simulink model "car_model_5_28_2023"  (R2022b)
settings: Solver=VariableStepAuto  StartTime=0.0  StopTime=15  RelTol=1e-3
values from neighbouring files (symbols this model uses):
  dZ = 0.295    [Startup.m]
  F0z = [0 0]    [Startup.m]
  phi = 45    [Startup.m]
  X = Reference_Signals.Chassis_Position.X.Data(:)    [Simulation_Data_Parse.m]    (also in Vehicle_Sim_Parse.m = Chassis_Signals.InertFrm.Cg.Disp.X.Data(:))
  Y = Reference_Signals.Chassis_Position.Y.Data(:)    [Simulation_Data_Parse.m]    (also in Vehicle_Sim_Parse.m = Chassis_Signals.InertFrm.Cg.Disp.Y.Data(:))
undefined symbols (not defined in the file or in its folder): chassis, DiscIntNeverNeededParam, driver, IMU_accel, IMU_gyro, IMU_mag, powertrain, psi, sensor, sim, sus, suspension, theta, trn, tvs, veh, VEH, whl, Xdot, Ydot, Z, Zdot
libraries: fl_lib x53, nesl_utility x15, vehdynlibtire x10, vehdynlibsuspension x8, EngineCoolingComponents_lib x5, autolibutils x5, sharedtransform x5, dspstat3 x2, simulink x2, slpidlib x2, shared6dof x2, sensorgpslib x1
(part 6 of 9)

== system car_model_5_28_2023/Vehicle Model/Suspension/MacPherson Suspension/Wheel  Adapter ==
  Wheels : Inport
  Bus Selector : BusSelector  OutputSignals=SuspFrame.Fx,SuspFrame.Fy
  Bus Selector1 : BusSelector  OutputSignals=SuspFrame.Re
  Bus Selector2 : BusSelector  OutputSignals=SuspFrame.Mx,SuspFrame.My,SuspFrame.Mz
  Bus Selector3 : BusSelector  OutputSignals=SuspFrame.z,SuspFrame.zdot
  Matrix Concatenate : Concatenate  NumInputs=3  Mode=Multidimensional array
  Reshape{,1..7} (8 alike) : Reshape  OutputDimensionality=Row vector (2-D)
  WhlFx : Outport  VectorParamsAs1DForOutWhenUnconnected=off
  WhlFy : Outport  Port=2  VectorParamsAs1DForOutWhenUnconnected=off
  z : Outport  Port=3  VectorParamsAs1DForOutWhenUnconnected=off
  zdot : Outport  Port=4  VectorParamsAs1DForOutWhenUnconnected=off
  M : Outport  Port=5  VectorParamsAs1DForOutWhenUnconnected=off
  Re : Outport  Port=6  VectorParamsAs1DForOutWhenUnconnected=off
  wires:
  Reshape7/1 -> WhlFy/1
  Reshape6/1 -> WhlFx/1
  Bus Selector/1 -> Reshape6/1  "<Fx>"
  Bus Selector/2 -> Reshape7/1  "<Fy>"
  Bus Selector3/1 -> Reshape/1  "<z>"
  Wheels/1 -> Bus Selector1/1, Bus Selector2/1, Bus Selector3/1, Bus Selector/1
  Bus Selector3/2 -> Reshape2/1  "<zdot>"
  Reshape2/1 -> zdot/1  "zdot"
  Bus Selector1/1 -> Reshape1/1  "<Re>"
  Reshape1/1 -> Re/1  "Re"
  Bus Selector2/1 -> Reshape3/1  "<Mx>"
  Bus Selector2/2 -> Reshape4/1  "<My>"
  Bus Selector2/3 -> Reshape5/1  "<Mz>"
  Reshape3/1 -> Matrix Concatenate/1
  Reshape4/1 -> Matrix Concatenate/2
  Reshape5/1 -> Matrix Concatenate/3
  Matrix Concatenate/1 -> M/1  "M"
  Reshape/1 -> z/1  "z"

== system car_model_5_28_2023/Vehicle Model/Suspension/Mapped Suspension/Steer Rate Adapter ==
  Veh : Inport
  Add : Sum
  Bus Selector3 : BusSelector  OutputSignals=BdyFrm.Cg.AngVel.r
  Constant : Constant  Value=zeros(1,4)
  Matrix Concatenate : Concatenate  NumInputs=3  Mode=Multidimensional array
  Matrix Concatenate1 : Concatenate  NumInputs=3  Mode=Multidimensional array
  Reshape2 : Reshape  OutputDimensionality=Row vector (2-D)
  Reshape3 : Reshape  OutputDimensionality=Row vector (2-D)
  Reshape4 : Reshape  OutputDimensionality=Row vector (2-D)
  Selector3 : Selector  InputPortWidth=1  IndexOptions=Index vector (dialog)  Indices=[1 1 1 1]  OutputSizes=1
  SteerRates : Constant  Value=zeros(1,4)
  AngVel : Outport  VectorParamsAs1DForOutWhenUnconnected=off
  wires:
  Reshape2/1 -> Matrix Concatenate1/1, Matrix Concatenate1/3, Matrix Concatenate1/2
  Constant/1 -> Reshape3/1
  Selector3/1 -> Reshape4/1
  Bus Selector3/1 -> Selector3/1  "<r>"
  Matrix Concatenate/1 -> Add/2
  SteerRates/1 -> Reshape2/1
  Reshape4/1 -> Matrix Concatenate/3
  Reshape3/1 -> Matrix Concatenate/2, Matrix Concatenate/1
  Matrix Concatenate1/1 -> Add/1
  Veh/1 -> Bus Selector3/1
  Add/1 -> AngVel/1  "AngVel"

== system car_model_5_28_2023/Vehicle Model/Suspension/Mapped Suspension/Vehicle Adapter ==
  Veh : Inport
  Bus Creator3 : BusCreator  Inputs=2
  Bus Selector1 : BusSelector  OutputSignals=InertFrm.FrntAxl.Lft.Disp.X,InertFrm.FrntAxl.Lft.Disp.Y,InertFrm.FrntAxl.Lft.Disp.Z,InertFrm.FrntAxl.Rght.Disp.X,InertFrm.FrntAxl.Rght.Disp.Y,InertFrm.FrntAxl.Rght.Disp.Z,InertFrm.RearAxl.Lft.Disp.X,InertFrm.RearAxl.Lft.Disp.Y,InertFrm.RearAxl.Lft.Disp.Z,InertFrm.RearAxl.Rght.Disp.X,InertFrm.RearAxl.Rght.Disp.Y,InertFrm.RearAxl.Rght.Disp.Z
  Bus Selector2 : BusSelector  OutputSignals=BdyFrm.FrntAxl.Lft.Vel.xdot,BdyFrm.FrntAxl.Lft.Vel.ydot,BdyFrm.FrntAxl.Lft.Vel.zdot,BdyFrm.FrntAxl.Rght.Vel.xdot,BdyFrm.FrntAxl.Rght.Vel.ydot,BdyFrm.FrntAxl.Rght.Vel.zdot,BdyFrm.RearAxl.Lft.Vel.xdot,BdyFrm.RearAxl.Lft.Vel.ydot,BdyFrm.RearAxl.Lft.Vel.zdot,BdyFrm.RearAxl.Rght.Vel.xdot,BdyFrm.RearAxl.Rght.Vel.ydot,BdyFrm.RearAxl.Rght.Vel.zdot
  Bus Selector3 : BusSelector  OutputSignals=InertFrm.FrntAxl.Lft.Vel.Xdot,InertFrm.FrntAxl.Lft.Vel.Ydot,InertFrm.FrntAxl.Lft.Vel.Zdot,InertFrm.FrntAxl.Rght.Vel.Xdot,InertFrm.FrntAxl.Rght.Vel.Ydot,InertFrm.FrntAxl.Rght.Vel.Zdot,InertFrm.RearAxl.Lft.Vel.Xdot,InertFrm.RearAxl.Lft.Vel.Ydot,InertFrm.RearAxl.Lft.Vel.Zdot,InertFrm.RearAxl.Rght.Vel.Xdot,InertFrm.RearAxl.Rght.Vel.Ydot,InertFrm.RearAxl.Rght.Vel.Zdot
  Inertial Frame CG to Axle Offset : Constant  Value=[zeros(2,4);dZ*ones(1,4)]
  Mux1 : Mux  Inputs=12
  Mux2 : Mux  Inputs=12
  Mux3 : Mux  Inputs=12
  Reshape : Reshape  OutputDimensionality=Customize  OutputDimensions=[3,4]
  Reshape1 : Reshape  OutputDimensionality=Customize  OutputDimensions=[3,4]
  Reshape2 : Reshape  OutputDimensionality=Customize  OutputDimensions=[3,4]
  Sum : Sum  Inputs=|+-
  VehSusp : Outport  VectorParamsAs1DForOutWhenUnconnected=off
  VehVbody : Outport  Port=2  VectorParamsAs1DForOutWhenUnconnected=off
  wires:
  Veh/1 -> Bus Selector3/1, Bus Selector2/1, Bus Selector1/1
  Reshape2/1 -> VehVbody/1  "V"
  Bus Creator3/1 -> VehSusp/1  "Veh"
  Reshape/1 -> Sum/1
  Bus Selector1/1 -> Mux2/1  "<X>"
  Bus Selector1/2 -> Mux2/2  "<Y>"
  Bus Selector1/3 -> Mux2/3  "<Z>"
  Bus Selector1/4 -> Mux2/4  "<X>"
  Bus Selector1/5 -> Mux2/5  "<Y>"
  Bus Selector1/6 -> Mux2/6  "<Z>"
  Bus Selector1/7 -> Mux2/7  "<X>"
  Bus Selector1/8 -> Mux2/8  "<Y>"
  Bus Selector1/9 -> Mux2/9  "<Z>"
  Bus Selector1/10 -> Mux2/10  "<X>"
  Bus Selector1/11 -> Mux2/11  "<Y>"
  Bus Selector1/12 -> Mux2/12  "<Z>"
  Bus Selector2/1 -> Mux1/1  "<xdot>"
  Bus Selector2/2 -> Mux1/2  "<ydot>"
  Bus Selector2/3 -> Mux1/3  "<zdot>"
  Bus Selector2/4 -> Mux1/4  "<xdot>"
  Bus Selector2/5 -> Mux1/5  "<ydot>"
  Bus Selector2/6 -> Mux1/6  "<zdot>"
  Bus Selector2/7 -> Mux1/7  "<xdot>"
  Bus Selector2/8 -> Mux1/8  "<ydot>"
  Bus Selector2/9 -> Mux1/9  "<zdot>"
  Bus Selector2/10 -> Mux1/10  "<xdot>"
  Bus Selector2/11 -> Mux1/11  "<ydot>"
  Bus Selector2/12 -> Mux1/12  "<zdot>"
  Mux1/1 -> Reshape2/1
  Mux2/1 -> Reshape/1
  Inertial Frame CG to Axle Offset/1 -> Sum/2
  Sum/1 -> Bus Creator3/1  "P"
  Mux3/1 -> Reshape1/1
  Bus Selector3/12 -> Mux3/12  "<Zdot>"
  Bus Selector3/11 -> Mux3/11  "<Ydot>"
  Bus Selector3/10 -> Mux3/10  "<Xdot>"
  Bus Selector3/9 -> Mux3/9  "<Zdot>"
  Bus Selector3/8 -> Mux3/8  "<Ydot>"
  Bus Selector3/7 -> Mux3/7  "<Xdot>"
  Bus Selector3/6 -> Mux3/6  "<Zdot>"
  Bus Selector3/5 -> Mux3/5  "<Ydot>"
  Bus Selector3/4 -> Mux3/4  "<Xdot>"
  Bus Selector3/3 -> Mux3/3  "<Zdot>"
  Bus Selector3/2 -> Mux3/2  "<Ydot>"
  Bus Selector3/1 -> Mux3/1  "<Xdot>"
  Reshape1/1 -> Bus Creator3/2  "V"

== system car_model_5_28_2023/Vehicle Model/Suspension/Mapped Suspension/Wheel  Adapter ==
  Wheels : Inport
  Bus Selector : BusSelector  OutputSignals=SuspFrame.Fx,SuspFrame.Fy
  Bus Selector1 : BusSelector  OutputSignals=SuspFrame.Re
  Bus Selector2 : BusSelector  OutputSignals=SuspFrame.Mx,SuspFrame.My,SuspFrame.Mz
  Bus Selector3 : BusSelector  OutputSignals=SuspFrame.z,SuspFrame.zdot
  Matrix Concatenate : Concatenate  NumInputs=3  Mode=Multidimensional array
  Reshape{,1..7} (8 alike) : Reshape  OutputDimensionality=Row vector (2-D)
  WhlFx : Outport  VectorParamsAs1DForOutWhenUnconnected=off
  WhlFy : Outport  Port=2  VectorParamsAs1DForOutWhenUnconnected=off
  z : Outport  Port=3  VectorParamsAs1DForOutWhenUnconnected=off
  zdot : Outport  Port=4  VectorParamsAs1DForOutWhenUnconnected=off
  M : Outport  Port=5  VectorParamsAs1DForOutWhenUnconnected=off
  Re : Outport  Port=6  VectorParamsAs1DForOutWhenUnconnected=off
  wires:
  Reshape7/1 -> WhlFy/1
  Reshape6/1 -> WhlFx/1
  Bus Selector/1 -> Reshape6/1  "<Fx>"
  Bus Selector/2 -> Reshape7/1  "<Fy>"
  Bus Selector3/1 -> Reshape/1  "<z>"
  Wheels/1 -> Bus Selector1/1, Bus Selector2/1, Bus Selector3/1, Bus Selector/1
  Bus Selector3/2 -> Reshape2/1  "<zdot>"
  Reshape2/1 -> zdot/1  "zdot"
  Bus Selector1/1 -> Reshape1/1  "<Re>"
  Reshape1/1 -> Re/1  "Re"
  Bus Selector2/1 -> Reshape3/1  "<Mx>"
  Bus Selector2/2 -> Reshape4/1  "<My>"
  Bus Selector2/3 -> Reshape5/1  "<Mz>"
  Reshape3/1 -> Matrix Concatenate/1
  Reshape4/1 -> Matrix Concatenate/2
  Reshape5/1 -> Matrix Concatenate/3
  Matrix Concatenate/1 -> M/1  "M"
  Reshape/1 -> z/1  "z"

== system car_model_5_28_2023/Vehicle Model/Vehicle/6DOF/Suspension to Chasiss Transforms ==
  VehFdbk : Inport
  Suspension : Inport  Port=2
  Add : Sum  Inputs=+-
  Add1 : Sum
  Bus Selector : BusSelector  OutputSignals=BdyFrm.Cg.Vel.xdot
  Bus Selector1 : BusSelector  OutputSignals=BdyFrm.Cg.DCM
  Bus Selector2 : BusSelector  OutputSignals=BdyFrm.Cg.Acc.xddot,BdyFrm.Cg.Vel.ydot,BdyFrm.Cg.AngVel.r,BdyFrm.Cg.Acc.yddot,BdyFrm.Cg.Vel.xdot,BdyFrm.Cg.AngVel.r
  Bus Selector3 : BusSelector  OutputSignals=Whl.z,Veh.F,Veh.M
  Bus Selector4 : BusSelector  OutputSignals=InertFrm.Cg.Ang.phi,InertFrm.Cg.Ang.theta,InertFrm.Cg.Ang.psi  OutputAsBus=on
  Bus Selector6 : BusSelector  OutputSignals=InertFrm.Geom.Disp.X,InertFrm.Geom.Disp.Y,InertFrm.Geom.Disp.Z  OutputAsBus=on
  Bus to Vector3 : BusToVector
  Bus to Vector5 : BusToVector
  Bushings : autolibutils/Cont LPF  wc=40*pi  AbsoluteTolerance=auto  aMode=2
  Downforce : MATLAB Function  TreatAsAtomicUnit=on
  Estimated Unsprung Mass Orientation : MATLAB Function  TreatAsAtomicUnit=on  mask{trackW=mean(2.*chassis.geometry.s), wheelB=sum(chassis.geometry.l)}
      mask prompts: trackW "Vehicle track width, trackW [m]:"; wheelB "Vehicle wheelbase, wheelB [m]:"
      mask help: This block converts wheel ground height information into estimates of vehicle pitch, roll angles and vertical height in order to help in the visualization 3DOF based simulations with changes in terrain. Note that the resulting signals are only used as a visualization aid and do not account for the physical affects of the vehicle interacting with variable terrain or changes in orientation.
  Product : Product
  Product1 : Product
  Sum : Sum  Inputs=|++
  Susp2Body : Subsystem
  Terminator6 : Terminator
  Unary Minus : UnaryMinus
  Unsprung Masses : Gain  Gain=sum(chassis.mass.m_unsprung)  Multiplication=Matrix(u*K)
  Vector Concatenate : Concatenate
  Vector Concatenate1 : Concatenate
  Vertical : Constant  Value=0
  FsB : Outport
  MsB : Outport  Port=2
  Fext : Outport  Port=3
  wires:
  Bus Selector6/1 -> Bus to Vector5/1
  Bus Selector3/2 -> Susp2Body/4(Fs)  "<F>"
  VehFdbk/1 -> Bus Selector2/1, Bus Selector/1, Bus Selector1/1, Bus Selector6/1, Bus Selector4/1
  Bus Selector3/3 -> Susp2Body/5(Ms)  "<M>"
  Bus to Vector3/1 -> Estimated Unsprung Mass Orientation/1(angleIn), Susp2Body/2(VehAng)
  Bus Selector1/1 -> Susp2Body/1(DCM)  "<DCM>"
  Bus to Vector5/1 -> Estimated Unsprung Mass Orientation/2(GemoXYZIn)
  Suspension/1 -> Bus Selector3/1
  Bus Selector4/1 -> Bus to Vector3/1
  Estimated Unsprung Mass Orientation/2(GeomXYZ) -> Terminator6/1
  Bus Selector3/1 -> Estimated Unsprung Mass Orientation/3(Ground)  "<z>"
  Estimated Unsprung Mass Orientation/1(angles) -> Susp2Body/3(SuspAng)
  Susp2Body/2(MsB) -> MsB/1
  Bushings/1 -> Unsprung Masses/1
  Vector Concatenate1/1 -> Bushings/1
  Unsprung Masses/1 -> Vector Concatenate/1
  Susp2Body/1(FsB) -> FsB/1
  Vector Concatenate/1 -> Unary Minus/1
  Vertical/1 -> Vector Concatenate/2
  Bus Selector2/2 -> Product/1  "<ydot>"
  Bus Selector2/3 -> Product/2  "<r>"
  Bus Selector2/5 -> Product1/1  "<xdot>"
  Bus Selector2/6 -> Product1/2  "<r>"
  Add/1 -> Vector Concatenate1/1
  Product/1 -> Add/2
  Product1/1 -> Add1/2
  Bus Selector2/4 -> Add1/1  "<yddot>"
  Add1/1 -> Vector Concatenate1/2
  Bus Selector2/1 -> Add/1  "<xddot>"
  Unary Minus/1 -> Sum/1
  Sum/1 -> Fext/1
  Downforce/1(y) -> Sum/2
  Bus Selector/1 -> Downforce/1(u)  "<xdot>"

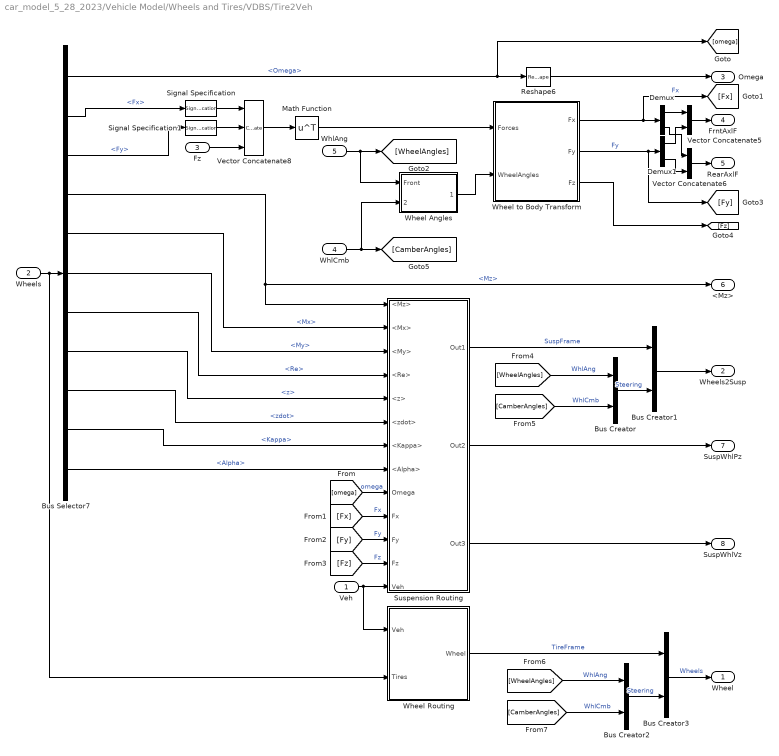
== system car_model_5_28_2023/Vehicle Model/Wheels and Tires/VDBS/Tire2Veh ==
  Veh : Inport
  Wheels : Inport  Port=2
  Fz : Inport  Port=3  PortDimensions=4
  WhlCmb : Inport  Port=4
  WhlAng : Inport  Port=5
  Bus Creator{,1..3} (4 alike) : BusCreator  Inputs=2
  Bus Selector7 : BusSelector  OutputSignals=Omega,Fx,Fy,Mz,Mx,My,Re,z,zdot,Kappa,Alpha
  Demux : Demux  Outputs=[2,2]
  Demux1 : Demux  Outputs=[2,2]
  Math Function : Math  Operator=transpose  SignedPower=on
  Reshape6 : Reshape  OutputDimensionality=Customize  OutputDimensions=[2,2]
  Signal Specification : SignalSpecification  Dimensions=4
  Signal Specification1 : SignalSpecification  Dimensions=4
  Suspension Routing : Subsystem
  Vector Concatenate5 : Concatenate  Mode=Multidimensional array  ConcatenateDimension=2
  Vector Concatenate6 : Concatenate  Mode=Multidimensional array  ConcatenateDimension=2
  Vector Concatenate8 : Concatenate  NumInputs=3  Mode=Multidimensional array  ConcatenateDimension=2
  Wheel Angles : Subsystem
  Wheel Routing : Subsystem
  Wheel to Body Transform : Subsystem
  Wheel : Outport  VectorParamsAs1DForOutWhenUnconnected=off
  Wheels2Susp : Outport  Port=2  VectorParamsAs1DForOutWhenUnconnected=off
  Omega : Outport  Port=3  VectorParamsAs1DForOutWhenUnconnected=off
  FrntAxlF : Outport  Port=4  VectorParamsAs1DForOutWhenUnconnected=off
  RearAxlF : Outport  Port=5  VectorParamsAs1DForOutWhenUnconnected=off
  <Mz> : Outport  Port=6  VectorParamsAs1DForOutWhenUnconnected=off
  SuspWhlPz : Outport  Port=7  VectorParamsAs1DForOutWhenUnconnected=off
  SuspWhlVz : Outport  Port=8  VectorParamsAs1DForOutWhenUnconnected=off
  wires:
  Fz/1 -> Vector Concatenate8/3
  Vector Concatenate6/1 -> RearAxlF/1
  Vector Concatenate8/1 -> Math Function/1
  Demux/2 -> Vector Concatenate6/1
  Demux1/2 -> Vector Concatenate6/2
  Demux/1 -> Vector Concatenate5/1
  Math Function/1 -> Wheel to Body Transform/1(Forces)
  Bus Selector7/2 -> Signal Specification/1  "<Fx>"
  Vector Concatenate5/1 -> FrntAxlF/1
  Wheels/1 -> Wheel Routing/2(Tires), Bus Selector7/1
  Reshape6/1 -> Omega/1
  Demux1/1 -> Vector Concatenate5/2
  Wheel Angles/1(Vehicle) -> Wheel to Body Transform/2(WheelAngles)
  Bus Selector7/1 -> [omega], Reshape6/1  "<Omega>"
  WhlAng/1 -> Wheel Angles/1(Front), [WheelAngles]
  Bus Selector7/4 -> <Mz>/1, Suspension Routing/1(<Mz>)  "<Mz>"
  Wheel to Body Transform/3(Fz) -> [Fz]
  WhlCmb/1 -> Wheel Angles/2(Camber), [CamberAngles]
  Bus Selector7/3 -> Signal Specification1/1  "<Fy>"
  Bus Selector7/5 -> Suspension Routing/2(<Mx>)  "<Mx>"
  Bus Selector7/6 -> Suspension Routing/3(<My>)  "<My>"
  Bus Selector7/7 -> Suspension Routing/4(<Re>)  "<Re>"
  [omega] -> Suspension Routing/9(Omega)  "omega"
  [Fx] -> Suspension Routing/10(Fx)  "Fx"
  Bus Selector7/8 -> Suspension Routing/5(<z>)  "<z>"
  [Fy] -> Suspension Routing/11(Fy)  "Fy"
  [Fz] -> Suspension Routing/12(Fz)  "Fz"
  Bus Selector7/9 -> Suspension Routing/6(<zdot>)  "<zdot>"
  Bus Selector7/10 -> Suspension Routing/7(<Kappa>)  "<Kappa>"
  Suspension Routing/2(Out2) -> SuspWhlPz/1
  Suspension Routing/3(Out3) -> SuspWhlVz/1
  [WheelAngles] -> Bus Creator/1  "WhlAng"
  Bus Creator1/1 -> Wheels2Susp/1
  Suspension Routing/1(Out1) -> Bus Creator1/1  "SuspFrame"
  [CamberAngles] -> Bus Creator/2  "WhlCmb"
  Bus Creator/1 -> Bus Creator1/2  "Steering"
  Bus Selector7/11 -> Suspension Routing/8(<Alpha>)  "<Alpha>"
  Wheel to Body Transform/1(Fx) -> [Fx], Demux/1  "Fx"
  Wheel to Body Transform/2(Fy) -> [Fy], Demux1/1  "Fy"
  Veh/1 -> Wheel Routing/1(Veh), Suspension Routing/13(Veh)
  Signal Specification/1 -> Vector Concatenate8/1
  Signal Specification1/1 -> Vector Concatenate8/2
  Wheel Routing/1(Wheel) -> Bus Creator3/1  "TireFrame"
  Bus Creator2/1 -> Bus Creator3/2  "Steering"
  [CamberAngles] -> Bus Creator2/2  "WhlCmb"
  Bus Creator3/1 -> Wheel/1  "Wheels"
  [WheelAngles] -> Bus Creator2/1  "WhlAng"

== system car_model_5_28_2023/Vehicle Model/Wheels and Tires/VDBS/Tires ==
  "DriveTorque " : Inport
  Brake Pedal : Inport  Port=2
  "r " : Inport  Port=3
  "Vx " : Inport  Port=4
  "Vy " : Inport  Port=5
  "Camber " : Inport  Port=6
  "Press " : Inport  Port=7
  "lambda " : Inport  Port=8
  "Gnd " : Inport  Port=9
  "FzSusp " : Inport  Port=10
  Fiala Tires : Subsystem  VariantControl=1
  Fiala Tires Vector : Subsystem  VariantControl=3
  MF Tires : Subsystem  VariantControl=0
  MF Tires Vector : Subsystem  VariantControl=2
  " Wheels" : Outport  VectorParamsAs1DForOutWhenUnconnected=off

== system car_model_5_28_2023/Vehicle Model/Wheels and Tires/VDBS/Veh2Tire ==
  r : Inport
  Axle : Inport  Port=2
  Brake Pedal : Inport  Port=3
  VehVel : Inport  Port=4
  WhlAng : Inport  Port=5
  WhlCmb : Inport  Port=6
  Demux4 : Demux
  Gain4 : Gain  Gain=[1;-1;1;-1]*0+1
  Mux1 : Mux
  Reshape{1..5} (5 alike) : Reshape
  Unary Minus : UnaryMinus
  Unary Minus1 : UnaryMinus
  Wheel Angles : Subsystem
  Wheel to Body Transform : Subsystem
  T : Outport  Unit=N*m  VectorParamsAs1DForOutWhenUnconnected=off
  P : Outport  Port=2  Unit=Pa  VectorParamsAs1DForOutWhenUnconnected=off
  psidot : Outport  Port=3  Unit=rad/s  VectorParamsAs1DForOutWhenUnconnected=off
  xdotAxle : Outport  Port=4  Unit=m/s  VectorParamsAs1DForOutWhenUnconnected=off
  ydotAxle : Outport  Port=5  Unit=m/s  VectorParamsAs1DForOutWhenUnconnected=off
  zdotAxle : Outport  Port=6  Unit=m/s  VectorParamsAs1DForOutWhenUnconnected=off
  Camber : Outport  Port=7  Unit=rad  VectorParamsAs1DForOutWhenUnconnected=off
  wires:
  Demux4/1 -> Mux1/1
  Demux4/4 -> Mux1/4
  Axle/1 -> Reshape4/1
  Wheel to Body Transform/1(xdotWheel) -> Reshape1/1  "Vx"
  Demux4/2 -> Mux1/2
  Wheel to Body Transform/2(ydotWheel) -> Reshape2/1  "Vy"
  WhlAng/1 -> Wheel Angles/1(steer)
  r/1 -> Unary Minus/1
  Demux4/3 -> Mux1/3
  Reshape3/1 -> Demux4/1
  Gain4/1 -> T/1
  Reshape4/1 -> Gain4/1
  VehVel/1 -> Wheel to Body Transform/1(VelVeh)
  Wheel to Body Transform/3(zdotWheel) -> Reshape5/1  "Vz"
  WhlCmb/1 -> Unary Minus1/1, Wheel Angles/2(camber)
  Unary Minus/1 -> psidot/1
  Wheel Angles/1(Vehicle) -> Wheel to Body Transform/2(WheelAngles)
  Reshape1/1 -> xdotAxle/1
  Reshape2/1 -> ydotAxle/1
  Reshape5/1 -> zdotAxle/1
  Unary Minus1/1 -> Camber/1
  Mux1/1 -> P/1
  Brake Pedal/1 -> Reshape3/1

== system car_model_5_28_2023/Vehicle Model/Wheels and Tires/VDBS/scale factors with friction ==
  lamda_mu_x : Inport
  lamda_mu_y : Inport  Port=2
  0 : Constant  Value=[zeros(1,numWheels)]  VectorParams1D=off
  1 : Constant  Value=[zeros(2,numWheels)]+1  VectorParams1D=off
  2 : Constant  Value=[zeros(1,numWheels)]+1  VectorParams1D=off
  Reshape : Reshape  OutputDimensionality=Row vector (2-D)  OutputDimensions=[1,numWheels]
  Reshape1 : Reshape  OutputDimensionality=Row vector (2-D)  OutputDimensions=[1,numWheels]
  Signal Specification3 : SignalSpecification  Unit=1
  Vector Concatenate : Concatenate  NumInputs=9  Mode=Multidimensional array
  ones : Constant  Value=[ones(6,numWheels)]  VectorParams1D=off
  ones1 : Constant  Value=[ones(9,numWheels)]  VectorParams1D=off
  ones2 : Constant  Value=ones(1,numWheels)  VectorParams1D=off
  ones3 : Constant  Value=[ones(5,numWheels)]  VectorParams1D=off
  lambdas : Outport  Unit=1  VectorParamsAs1DForOutWhenUnconnected=off
  wires:
  lamda_mu_y/1 -> Reshape1/1
  lamda_mu_x/1 -> Reshape/1
  ones2/1 -> Vector Concatenate/1  "lambda_Fz0"
  Vector Concatenate/1 -> Signal Specification3/1
  ones/1 -> Vector Concatenate/9
  0/1 -> Vector Concatenate/4  "lamda_mu_V"
  Reshape1/1 -> Vector Concatenate/3
  Reshape/1 -> Vector Concatenate/2
  Signal Specification3/1 -> lambdas/1
  1/1 -> Vector Concatenate/8  "lam_Vykappa"
  ones1/1 -> Vector Concatenate/5
  2/1 -> Vector Concatenate/6  "lam_Vy"
  ones3/1 -> Vector Concatenate/7

== system car_model_5_28_2023/Vehicle Model/Powertrain/Motor Cooling Loop/Motor FL/Sensor ==
  PS-Simulink Converter : nesl_utility/PS-Simulink Converter  PhysicalDomain=network_engine_domain  SubClassName=ps_output  LeftPortType=input  RightPortType=output  PseudoPeriodic=off  Frequencies=[]  VectorFormat=1-D array  Unit=1  AffineConversion=off
  Temperature Sensor : fl_lib/Thermal/Thermal Sensors/Temperature Sensor
  Thermal Reference : fl_lib/Thermal/Thermal Elements/Thermal Reference
  A : PMIOPort  Side=Left
  tag scope: MotorFL=global
  wires:
  PS-Simulink Converter/1 -> [MotorFL]
  connections:
  Temperature Sensor/LConn1 -- A/RConn1
  Temperature Sensor/RConn2 -- PS-Simulink Converter/LConn1
  Thermal Reference/LConn1 -- Temperature Sensor/RConn1

== system car_model_5_28_2023/Vehicle Model/Powertrain/Motor Cooling Loop/Motor FR/Sensor ==
  PS-Simulink Converter : nesl_utility/PS-Simulink Converter  PhysicalDomain=network_engine_domain  SubClassName=ps_output  LeftPortType=input  RightPortType=output  PseudoPeriodic=off  Frequencies=[]  VectorFormat=1-D array  Unit=1  AffineConversion=off
  Temperature Sensor : fl_lib/Thermal/Thermal Sensors/Temperature Sensor
  Thermal Reference : fl_lib/Thermal/Thermal Elements/Thermal Reference
  A : PMIOPort  Side=Left
  tag scope: MotorFR=global
  wires:
  PS-Simulink Converter/1 -> [MotorFR]
  connections:
  Temperature Sensor/LConn1 -- A/RConn1
  Temperature Sensor/RConn2 -- PS-Simulink Converter/LConn1
  Thermal Reference/LConn1 -- Temperature Sensor/RConn1

== system car_model_5_28_2023/Vehicle Model/Powertrain/Motor Cooling Loop/Motor RL/Sensor ==
  PS-Simulink Converter : nesl_utility/PS-Simulink Converter  PhysicalDomain=network_engine_domain  SubClassName=ps_output  LeftPortType=input  RightPortType=output  PseudoPeriodic=off  Frequencies=[]  VectorFormat=1-D array  Unit=1  AffineConversion=off
  Temperature Sensor : fl_lib/Thermal/Thermal Sensors/Temperature Sensor
  Thermal Reference : fl_lib/Thermal/Thermal Elements/Thermal Reference
  A : PMIOPort  Side=Left
  tag scope: MotorRL=global
  wires:
  PS-Simulink Converter/1 -> [MotorRL]
  connections:
  Temperature Sensor/LConn1 -- A/RConn1
  Temperature Sensor/RConn2 -- PS-Simulink Converter/LConn1
  Thermal Reference/LConn1 -- Temperature Sensor/RConn1

== system car_model_5_28_2023/Vehicle Model/Powertrain/Motor Cooling Loop/Motor RR/Sensor ==
  PS-Simulink Converter : nesl_utility/PS-Simulink Converter  PhysicalDomain=network_engine_domain  SubClassName=ps_output  LeftPortType=input  RightPortType=output  PseudoPeriodic=off  Frequencies=[]  VectorFormat=1-D array  Unit=1  AffineConversion=off
  Temperature Sensor : fl_lib/Thermal/Thermal Sensors/Temperature Sensor
  Thermal Reference : fl_lib/Thermal/Thermal Elements/Thermal Reference
  A : PMIOPort  Side=Left
  tag scope: MotorRR=global
  wires:
  PS-Simulink Converter/1 -> [MotorRR]
  connections:
  Temperature Sensor/LConn1 -- A/RConn1
  Temperature Sensor/RConn2 -- PS-Simulink Converter/LConn1
  Thermal Reference/LConn1 -- Temperature Sensor/RConn1

== system car_model_5_28_2023/Vehicle Model/Suspension/Double Wishbone Suspension/Steering Adapter/Steering Model ==
  steering_angle : Inport  OutMin=-130  OutMax=130  OutDataTypeStr=double  LockScale=on
  1-D Lookup Table : Lookup_n-D  NumberOfTableDimensions=1  BreakpointsForDimension1=suspension.steering.theta_sweep  Table=suspension.steering.theta_left  InterpMethod=Cubic spline  InternalRulePriority=Speed  RndMeth=Simplest
  1-D Lookup Table1 : Lookup_n-D  NumberOfTableDimensions=1  BreakpointsForDimension1=suspension.steering.theta_sweep  Table=suspension.steering.theta_right  InterpMethod=Cubic spline  InternalRulePriority=Speed  RndMeth=Simplest
  Mux : Mux  Inputs=2
  steering_angles : Outport  OutDataTypeStr=double  LockScale=on
  wires:
  1-D Lookup Table/1 -> Mux/1
  Mux/1 -> steering_angles/1  "steering_angles"
  1-D Lookup Table1/1 -> Mux/2
  steering_angle/1 -> 1-D Lookup Table1/1, 1-D Lookup Table/1

== system car_model_5_28_2023/Vehicle Model/Suspension/Kinematics and Compliance Independent Suspension/Calculate dynamic track width from lateral wheel center displacement change/Front Track Calculation ==
  dWhlY : Inport
  sign : Inport  Port=2
  Abs : Abs  ZeroCross=off  SaturateOnIntegerOverflow=off
  Abs1 : Abs  ZeroCross=off  SaturateOnIntegerOverflow=off
  Add : Sum  Inputs=+++
  Front Left select : Selector  InputPortWidth=4  IndexOptions=Index vector (dialog)  Indices=1  OutputSizes=1
  Front Left select1 : Selector  InputPortWidth=4  IndexOptions=Index vector (dialog)  Indices=1  OutputSizes=1
  Front Right select : Selector  InputPortWidth=4  IndexOptions=Index vector (dialog)  Indices=2  OutputSizes=1
  Front Right select1 : Selector  InputPortWidth=4  IndexOptions=Index vector (dialog)  Indices=2  OutputSizes=1
  Front Track : Constant  Value=w(1)
  Product : Product
  Product1 : Product
  w_front : Outport
  wires:
  Front Track/1 -> Add/1
  Front Left select/1 -> Abs/1
  Front Right select/1 -> Abs1/1
  sign/1 -> Front Right select1/1, Front Left select1/1
  Product/1 -> Add/2
  Front Left select1/1 -> Product/2
  Abs1/1 -> Product1/1
  Abs/1 -> Product/1
  Product1/1 -> Add/3
  Front Right select1/1 -> Product1/2
  Add/1 -> w_front/1
  dWhlY/1 -> Front Right select/1, Front Left select/1

== system car_model_5_28_2023/Vehicle Model/Suspension/Kinematics and Compliance Independent Suspension/Calculate dynamic track width from lateral wheel center displacement change/Rear Track Calculation ==
  dWhlY : Inport
  sign : Inport  Port=2
  Abs2 : Abs  ZeroCross=off  SaturateOnIntegerOverflow=off
  Abs3 : Abs  ZeroCross=off  SaturateOnIntegerOverflow=off
  Add1 : Sum  Inputs=+++
  Product2 : Product
  Product3 : Product
  Rear Left select : Selector  InputPortWidth=4  IndexOptions=Index vector (dialog)  Indices=3  OutputSizes=1
  Rear Left select1 : Selector  InputPortWidth=4  IndexOptions=Index vector (dialog)  Indices=3  OutputSizes=1
  Rear Right select : Selector  InputPortWidth=4  IndexOptions=Index vector (dialog)  Indices=4  OutputSizes=1
  Rear Right select1 : Selector  InputPortWidth=4  IndexOptions=Index vector (dialog)  Indices=4  OutputSizes=1
  Rear Track : Constant  Value=w(2)
  w_rear : Outport
  wires:
  Product2/1 -> Add1/2
  Abs2/1 -> Product2/1
  Rear Left select/1 -> Abs2/1
  Rear Left select1/1 -> Product2/2
  Rear Right select1/1 -> Product3/2
  Abs3/1 -> Product3/1
  dWhlY/1 -> Rear Left select/1, Rear Right select/1
  sign/1 -> Rear Right select1/1, Rear Left select1/1
  Rear Right select/1 -> Abs3/1
  Rear Track/1 -> Add1/1
  Product3/1 -> Add1/3
  Add1/1 -> w_rear/1

== system car_model_5_28_2023/Vehicle Model/Vehicle/6DOF/Suspension to Chasiss Transforms/Susp2Body ==
  DCM : Inport
  VehAng : Inport  Port=2
  SuspAng : Inport  Port=3
  Fs : Inport  Port=4  Partition=on  PartitionDimension=2  PartitionWidth=1  PartitionOffset=0
  Ms : Inport  Port=5  Partition=on  PartitionDimension=2  PartitionWidth=1  PartitionOffset=0
  For Each : ForEach  DisableCoverage=on
  Inertial to Body : Product  Multiplication=Matrix(*)  InputSameDT=on  SaturateOnIntegerOverflow=on  OutDataTypeStr=Inherit: Same as first input
  Inertial to Body1 : Product  Multiplication=Matrix(*)  InputSameDT=on  SaturateOnIntegerOverflow=on  OutDataTypeStr=Inherit: Same as first input
  Reshape : Reshape
  Reshape1 : Reshape
  Rotation Angles to Direction Cosine Matrix : sharedtransform/Rotation Angles to Direction Cosine Matrix  rotationOrder=ZYX  aMode=2
  Selector : Selector  InputPortWidth=3  IndexOptions=Index vector (dialog)  Indices=[3 2 1]  OutputSizes=1
  Selector1 : Selector  InputPortWidth=3  IndexOptions=Index vector (dialog)  Indices=[1 2]  OutputSizes=1
  Selector2 : Selector  InputPortWidth=3  IndexOptions=Index vector (dialog)  Indices=[3]  OutputSizes=1
  Transpose : Math  Operator=transpose  SignedPower=on
  Unary Minus : UnaryMinus
  Vector Concatenate : Concatenate
  "transform to Inertial axes " : shared6dof/6DOF (Euler Angles)/transform to Inertial axes   SystemSampleTime=-1  VariantActivationTime=update diagram  Latency=0  AutoFrameSizeCalculation=off
  transform to Inertial axes 1 : shared6dof/6DOF (Euler Angles)/transform to Inertial axes   SystemSampleTime=-1  VariantActivationTime=update diagram  Latency=0  AutoFrameSizeCalculation=off
  FsB : Outport  ConcatenationDimension=2  VectorParamsAs1DForOutWhenUnconnected=off
  MsB : Outport  Port=2  ConcatenationDimension=2  VectorParamsAs1DForOutWhenUnconnected=off
  wires:
  Reshape/1 -> Inertial to Body/2
  Inertial to Body/1 -> FsB/1
  SuspAng/1 -> Unary Minus/1
  Selector/1 -> Rotation Angles to Direction Cosine Matrix/1
  Fs/1 -> "transform to Inertial axes "/1
  Transpose/1 -> transform to Inertial axes 1/2, "transform to Inertial axes "/2
  Rotation Angles to Direction Cosine Matrix/1 -> Transpose/1
  "transform to Inertial axes "/1 -> Reshape/1
  transform to Inertial axes 1/1 -> Reshape1/1
  Inertial to Body1/1 -> MsB/1
  Reshape1/1 -> Inertial to Body1/2
  DCM/1 -> Inertial to Body1/1, Inertial to Body/1
  Ms/1 -> transform to Inertial axes 1/1
  VehAng/1 -> Selector2/1
  Unary Minus/1 -> Selector1/1
  Selector1/1 -> Vector Concatenate/1
  Vector Concatenate/1 -> Selector/1
  Selector2/1 -> Vector Concatenate/2

== system car_model_5_28_2023/Vehicle Model/Wheels and Tires/VDBS/Tire2Veh/Suspension Routing ==
  <Mz> : Inport
  <Mx> : Inport  Port=2
  <My> : Inport  Port=3
  <Re> : Inport  Port=4
  <z> : Inport  Port=5
  <zdot> : Inport  Port=6
  <Kappa> : Inport  Port=7
  <Alpha> : Inport  Port=8
  Omega : Inport  Port=9
  Fx : Inport  Port=10
  Fy : Inport  Port=11
  Fz : Inport  Port=12
  Veh : Inport  Port=13
  Bus Creator : BusCreator  Inputs=13
  Bus Selector3 : BusSelector  OutputSignals=InertFrm.FrntAxl.Lft.Disp.Z,InertFrm.FrntAxl.Rght.Disp.Z,InertFrm.RearAxl.Lft.Disp.Z,InertFrm.RearAxl.Rght.Disp.Z
  Bus Selector4 : BusSelector  OutputSignals=BdyFrm.FrntAxl.Lft.Disp.z,BdyFrm.FrntAxl.Rght.Disp.z,BdyFrm.RearAxl.Lft.Disp.z,BdyFrm.RearAxl.Rght.Disp.z
  Reshape : Reshape  OutputDimensionality=Row vector (2-D)
  Reshape1 : Reshape  OutputDimensionality=Row vector (2-D)
  Subtract : Sum  Inputs=--+
  Unary Minus1 : UnaryMinus
  Unary Minus2 : UnaryMinus
  Vector Concatenate3 : Concatenate  NumInputs=4
  Vector Concatenate4 : Concatenate  NumInputs=4
  Out1 : Outport  VectorParamsAs1DForOutWhenUnconnected=off
  Out2 : Outport  Port=2  VectorParamsAs1DForOutWhenUnconnected=off
  Out3 : Outport  Port=3  VectorParamsAs1DForOutWhenUnconnected=off
  wires:
  <Re>/1 -> Bus Creator/8
  Unary Minus1/1 -> Bus Creator/10, Subtract/1, Reshape/1  "z"
  Fz/1 -> Bus Creator/4
  <zdot>/1 -> Unary Minus2/1
  <Mz>/1 -> Bus Creator/7
  Unary Minus2/1 -> Bus Creator/11, Reshape1/1  "zdot"
  <z>/1 -> Unary Minus1/1
  Bus Creator/1 -> Out1/1
  Fy/1 -> Bus Creator/3
  Omega/1 -> Bus Creator/1  "Omega"
  Fx/1 -> Bus Creator/2
  Reshape1/1 -> Out3/1
  <Kappa>/1 -> Bus Creator/12
  Reshape/1 -> Out2/1
  <Mx>/1 -> Bus Creator/5
  <My>/1 -> Bus Creator/6
  <Alpha>/1 -> Bus Creator/13
  Veh/1 -> Bus Selector3/1, Bus Selector4/1
  Bus Selector3/4 -> Vector Concatenate3/4  "<Z>"
  Subtract/1 -> Bus Creator/9  "dz"
  Bus Selector4/1 -> Vector Concatenate4/1  "<z>"
  Bus Selector3/1 -> Vector Concatenate3/1  "<Z>"
  Vector Concatenate3/1 -> Subtract/3
  Vector Concatenate4/1 -> Subtract/2
  Bus Selector4/2 -> Vector Concatenate4/2  "<z>"
  Bus Selector3/3 -> Vector Concatenate3/3  "<Z>"
  Bus Selector3/2 -> Vector Concatenate3/2  "<Z>"
  Bus Selector4/4 -> Vector Concatenate4/4  "<z>"
  Bus Selector4/3 -> Vector Concatenate4/3  "<z>"

== system car_model_5_28_2023/Vehicle Model/Wheels and Tires/VDBS/Tire2Veh/Wheel Angles ==
  Front : Inport
  Camber : Inport  Port=2
  Constant : Constant  Value=zeros(4,1)
  Reshape : Reshape  OutputDimensionality=Row vector (2-D)
  Reshape1 : Reshape  OutputDimensionality=Row vector (2-D)
  Reshape2 : Reshape  OutputDimensionality=Row vector (2-D)
  Vector Concatenate3 : Concatenate  NumInputs=3  Mode=Multidimensional array
  Vehicle : Outport  VectorParamsAs1DForOutWhenUnconnected=off
  wires:
  Reshape/1 -> Vector Concatenate3/3
  Reshape2/1 -> Vector Concatenate3/2
  Vector Concatenate3/1 -> Vehicle/1
  Reshape1/1 -> Vector Concatenate3/1
  Front/1 -> Reshape/1
  Camber/1 -> Reshape1/1
  Constant/1 -> Reshape2/1

== system car_model_5_28_2023/Vehicle Model/Wheels and Tires/VDBS/Tire2Veh/Wheel Routing ==
  Veh : Inport
  Tires : Inport  Port=2
  Bus Creator : BusCreator  Inputs=14
  Bus Selector : BusSelector  OutputSignals=Omega,Fx,Fy,Fz,GndFz,Mx,My,Mz,Re,z,zdot,Kappa,Alpha
  Bus Selector3 : BusSelector  OutputSignals=InertFrm.FrntAxl.Lft.Disp.Z,InertFrm.FrntAxl.Rght.Disp.Z,InertFrm.RearAxl.Lft.Disp.Z,InertFrm.RearAxl.Rght.Disp.Z
  Bus Selector4 : BusSelector  OutputSignals=BdyFrm.FrntAxl.Lft.Disp.z,BdyFrm.FrntAxl.Rght.Disp.z,BdyFrm.RearAxl.Lft.Disp.z,BdyFrm.RearAxl.Rght.Disp.z
  Subtract : Sum  Inputs=-+-
  Vector Concatenate3 : Concatenate  NumInputs=4
  Vector Concatenate4 : Concatenate  NumInputs=4
  Wheel : Outport  VectorParamsAs1DForOutWhenUnconnected=off
  wires:
  Bus Selector4/3 -> Vector Concatenate4/3  "<z>"
  Bus Selector4/4 -> Vector Concatenate4/4  "<z>"
  Bus Selector3/2 -> Vector Concatenate3/2  "<Z>"
  Bus Selector3/3 -> Vector Concatenate3/3  "<Z>"
  Bus Selector4/2 -> Vector Concatenate4/2  "<z>"
  Vector Concatenate4/1 -> Subtract/2
  Vector Concatenate3/1 -> Subtract/3
  Bus Selector3/1 -> Vector Concatenate3/1  "<Z>"
  Bus Selector4/1 -> Vector Concatenate4/1  "<z>"
  Subtract/1 -> Bus Creator/10  "dz"
  Bus Selector3/4 -> Vector Concatenate3/4  "<Z>"
  Veh/1 -> Bus Selector4/1, Bus Selector3/1
  Bus Selector/13 -> Bus Creator/14  "<Alpha>"
  Bus Selector/7 -> Bus Creator/7  "<My>"
  Bus Selector/6 -> Bus Creator/6  "<Mx>"
  Bus Selector/12 -> Bus Creator/13  "<Kappa>"
  Bus Selector/2 -> Bus Creator/2  "<Fx>"
  Bus Selector/1 -> Bus Creator/1  "<Omega>"
  Bus Selector/3 -> Bus Creator/3  "<Fy>"
  Bus Creator/1 -> Wheel/1
  Bus Selector/11 -> Bus Creator/12  "<zdot>"
  Bus Selector/8 -> Bus Creator/8  "<Mz>"
  Bus Selector/4 -> Bus Creator/4  "<Fz>"
  Bus Selector/10 -> Bus Creator/11, Subtract/1  "<z>"
  Tires/1 -> Bus Selector/1  "TireFrame"
  Bus Selector/9 -> Bus Creator/9  "<Re>"
  Bus Selector/5 -> Bus Creator/5  "<GndFz>"

== system car_model_5_28_2023/Vehicle Model/Wheels and Tires/VDBS/Tire2Veh/Wheel to Body Transform ==
  Forces : Inport  PortDimensions=[3,1]  Partition=on  PartitionDimension=2  PartitionWidth=1  PartitionOffset=0
  WheelAngles : Inport  Port=2  Partition=on  PartitionDimension=2  PartitionWidth=1  PartitionOffset=0
  Constant : Constant  Value=[pi;0;0]
  Demux1 : Demux  Outputs=3
  Divide1 : Product  Inputs=***  Multiplication=Matrix(*)
  For Each : ForEach  DisableCoverage=on
  Rotation Angles to Direction Cosine Matrix : sharedtransform/Rotation Angles to Direction Cosine Matrix  rotationOrder=ZYX  aMode=2
  Rotation Angles to Direction Cosine Matrix1 : sharedtransform/Rotation Angles to Direction Cosine Matrix  rotationOrder=ZYX  aMode=2
  Selector : Selector  InputPortWidth=3  IndexOptions=Index vector (dialog)  Indices=[3 2 1]  OutputSizes=1
  Selector1 : Selector  InputPortWidth=3  IndexOptions=Index vector (dialog)  Indices=[3 2 1]  OutputSizes=1
  Transpose : Math  Operator=transpose
  Fx : Outport  ConcatenationDimension=1  VectorParamsAs1DForOutWhenUnconnected=off
  Fy : Outport  Port=2  ConcatenationDimension=1  VectorParamsAs1DForOutWhenUnconnected=off
  Fz : Outport  Port=3  ConcatenationDimension=1  VectorParamsAs1DForOutWhenUnconnected=off
  wires:
  Demux1/1 -> Fx/1
  Demux1/2 -> Fy/1
  Demux1/3 -> Fz/1
  Rotation Angles to Direction Cosine Matrix/1 -> Transpose/1
  Forces/1 -> Divide1/3
  WheelAngles/1 -> Selector/1
  Selector/1 -> Rotation Angles to Direction Cosine Matrix/1
  Rotation Angles to Direction Cosine Matrix1/1 -> Divide1/2
  Divide1/1 -> Demux1/1
  Selector1/1 -> Rotation Angles to Direction Cosine Matrix1/1
  Constant/1 -> Selector1/1
  Transpose/1 -> Divide1/1
